simulink model "calcula_velocidade"  (R2012b)
settings: Solver=FixedStepDiscrete  StartTime=0  StopTime=final_time  FixedStep=step_size  MaxStep=1e-4  RelTol=1e-3
libraries: simulink x3, Encoder x1
settings Model: Creator=h3now  LastModifiedBy=h3now
settings DataIOCC: ExternalInput=[time, Hall1, Hall2, Hall3]  LimitDataPoints=off  LoadExternalInput=on  SaveTime=off

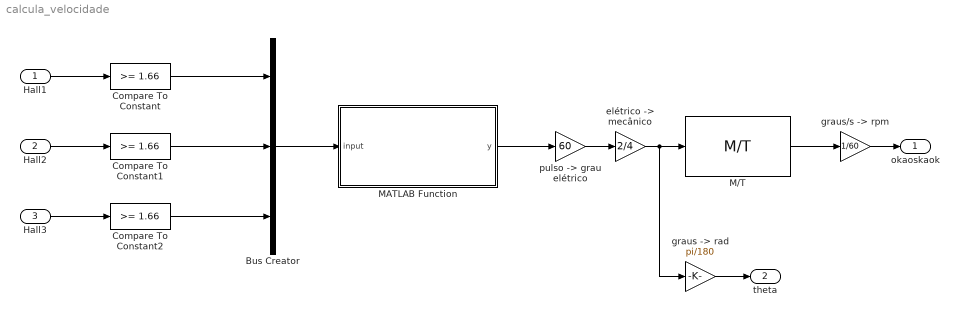
== system calcula_velocidade ==
  Hall1 : Inport
  Hall2 : Inport  Port=2
  Hall3 : Inport  Port=3
  Bus Creator : BusCreator  Inputs=3
  Compare To Constant : simulink/Logic and Bit Operations/Compare To Constant  relop=>=  const=1.66  OutDataTypeStr=uint8
  Compare To Constant1 : simulink/Logic and Bit Operations/Compare To Constant  relop=>=  const=1.66  OutDataTypeStr=uint8
  Compare To Constant2 : simulink/Logic and Bit Operations/Compare To Constant  relop=>=  const=1.66  OutDataTypeStr=uint8
  M/T : Encoder/M//T  Ts=0.01
  MATLAB Function : MATLAB Function  TreatAsAtomicUnit=on
  "elétrico -> mecânico" : Gain  Gain=2/4
  "graus -> rad" : Gain  Gain=pi/180
  "graus/s -> rpm" : Gain  Gain=1/60
  "pulso -> grau elétrico" : Gain  Gain=60
  okaoskaok : Outport
  theta : Outport  Port=2
  wires:
  Bus Creator/1 -> MATLAB Function/1(input)
  Hall1/1 -> Compare To Constant/1
  Hall2/1 -> Compare To Constant1/1
  Compare To Constant/1 -> Bus Creator/1
  Compare To Constant1/1 -> Bus Creator/2
  Compare To Constant2/1 -> Bus Creator/3
  MATLAB Function/1(y) -> "pulso -> grau elétrico"/1
  "pulso -> grau elétrico"/1 -> "elétrico -> mecânico"/1
  "elétrico -> mecânico"/1 -> "graus -> rad"/1, M/T/1
  M/T/1 -> "graus/s -> rpm"/1
  Hall3/1 -> Compare To Constant2/1
  "graus/s -> rpm"/1 -> okaoskaok/1
  "graus -> rad"/1 -> theta/1

== matlab function calcula_velocidade/MATLAB Function ==
  data: y output; input input
function y = state_machine(input)
%#codegen

% Initializing persistent variables.
persistent theta;
persistent state;
if isempty(theta)
    % 'theta' stores the angular position.
    theta = 0; 
    
    % check starting state and store it in 'state'.
    if isequal(input, [0,0,1]')
        state = 0;
    elseif isequal(input, [1,0,1]')
        state = 1;
    elseif isequal(input, [1,0,0]')
        state = 2;
    elseif isequal(input, [1,1,0]')
        state = 3;
    elseif isequal(input, [0,1,0]')
        state = 4;
    elseif isequal(input, [0,1,1]')
        state = 5;
    else
        state = -1;
    end
        
end

% State machine.
switch state
    case 0
        % keep state.
        if isequal(input,[0,0,1]')
        % go to next state.
        elseif isequal(input,[1,0,1]')
            state = 1;
            theta = theta + 1;
        % go to previous state.
        elseif isequal(input,[0,1,1]')
            state = 5;
            theta = theta - 1;
        % go to error state.
        else
            state = -1;
        end
        
    case 1
        % keep state.
        if isequal(input,[1,0,1]')
        % go to next state.
        elseif isequal(input,[1,0,0]')
            state = 2;
            theta = theta + 1;
        % go to previous state.
        elseif isequal(input,[0,0,1]')
            state = 0;
            theta = theta - 1;
        % go to error state.
        else
            state = -1;
        end
        
    case 2
        % keep state.
        if isequal(input,[1,0,0]')
        % go to next state.
        elseif isequal(input,[1,1,0]')
            state = 3;
            theta = theta + 1;
        % go to previous state.
        elseif isequal(input,[1,0,1]')
            state = 1;
            theta = theta - 1;
        % go to error state.
        else
            state = -1;
        end
        
    case 3
        % keep state.
        if isequal(input,[1,1,0]')
        % go to next state.
        elseif isequal(input,[0,1,0]')
            state = 4;
            theta = theta + 1;
        % go to previous state.
        elseif isequal(input,[1,0,0]')
            state = 2;
            theta = theta - 1;
        % go to error state.
        else
            state = -1;
        end
        
    case 4
        % keep state.
        if isequal(input,[0,1,0]')
        % go to next state.
        elseif isequal(input,[0,1,1]')
            state = 5;
            theta = theta + 1;
        % go to previous state.
        elseif isequal(input,[1,1,0]')
            state = 3;
            theta = theta - 1;
        % go to error state.
        else
            state = -1;
        end
        
    case 5
        % keep state.
        if isequal(input,[0,1,1]')
        % go to next state.
        elseif isequal(input,[0,0,1]')
            state = 0;
            theta = theta + 1;
        % go to previous state.
        elseif isequal(input,[0,1,0]')
            state = 4;
            theta = theta - 1;
        % go to error state.
        else
            state = -1;
        end
            
end

% Output
y = theta;
